simulink model "KalmanObserver_R2021b"  (R2021b)
settings: Solver=ode1  StartTime=0.0  StopTime=10  FixedStep=0.01  RelTol=1e-3
libraries: TcTargetLib x10
settings Model: SimulationMode=external  NumberOfSteps=50  PacingRate=0.280000  Creator=ATLabor  LastModifiedBy=Mergin
settings OptimizationCC: LocalBlockOutputs=off
settings RTWCC: Description=TwinCAT GRT Target  SystemTargetFile=TwinCatGrt.tlc  GenCodeOnly=on  TemplateMakefile=tcgrt_msbuild.tmf  TargetLang=C++
settings STFCustomTargetCC: TargetLangStandard=C++11 (ISO)  CombineOutputUpdateFcns=on  CPPClassGenCompliant=on  GRTInterface=off  SystemTargetFile=TwinCatGrt.tlc
settings GRTTargetCC: TargetLangStandard=C++11 (ISO)  ParMdlRefBuildCompliant=off  CompOptLevelCompliant=off  ConcurrentExecutionCompliant=off  MatFileLogging=off  UseToolchainInfoCompliant=off  ExtModeMexFile=TcExtModeClient

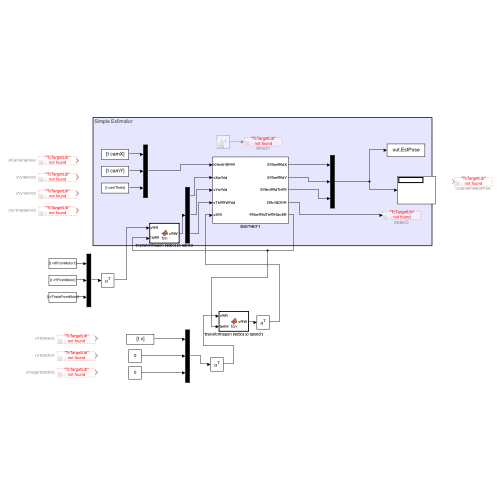
[thumbnail: Simulink's stored preview of the top-level diagram]
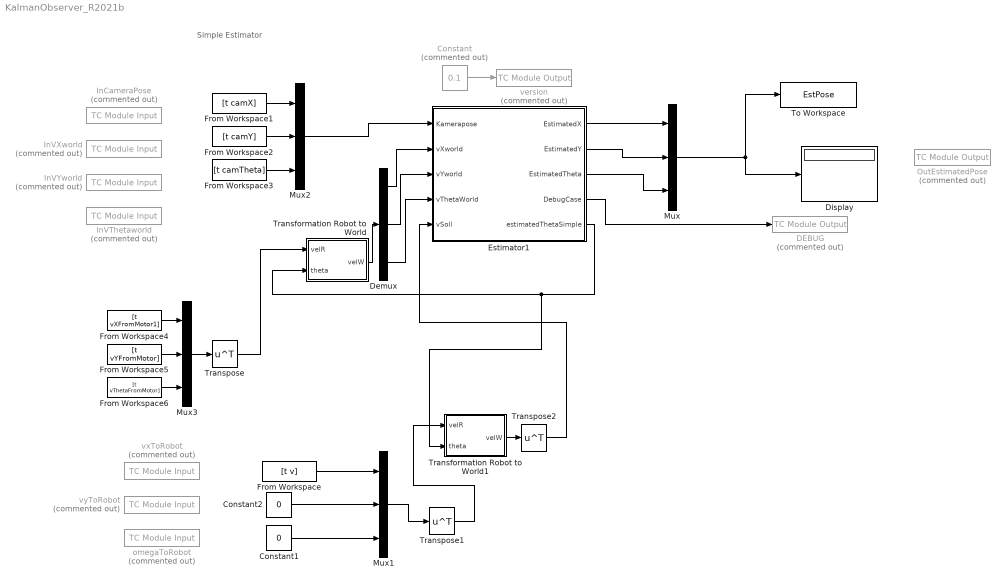
== system KalmanObserver_R2021b ==
  note: Simple Estimator
  Constant : Constant  Commented=on  Value=0.1
  Constant1 : Constant  Value=0
  Constant2 : Constant  Value=0
  DEBUG : TcTargetLib/TC Module Output  Commented=on  PortDataType=double  PortDim=1  SampleTime=-1  CodeGenConnectType=DataArea (OutputSrc)  DataTypeOverride=off
  Demux : Demux  Outputs=3
  Display : Display
  Estimator1 : Subsystem
  From Workspace : FromWorkspace  VariableName=[t v]  SampleTime=10e-3  OutputAfterFinalValue=Setting to zero
  From Workspace1 : FromWorkspace  VariableName=[t camX]  OutputAfterFinalValue=Holding final value
  From Workspace2 : FromWorkspace  VariableName=[t camY]  OutputAfterFinalValue=Holding final value
  From Workspace3 : FromWorkspace  VariableName=[t camTheta]  OutputAfterFinalValue=Holding final value
  From Workspace4 : FromWorkspace  VariableName=[t vXFromMotor1]  OutputAfterFinalValue=Setting to zero
  From Workspace5 : FromWorkspace  VariableName=[t vYFromMotor]  OutputAfterFinalValue=Setting to zero
  From Workspace6 : FromWorkspace  VariableName=[t vThetaFromMotor]  OutputAfterFinalValue=Setting to zero
  InCameraPose : TcTargetLib/TC Module Input  Commented=on  PortDataType=double  PortDim=3  Value=[0 0 0]  SampleTime=-1  CodeGenConnectType=DataArea (InputDst)  DataTypeOverride=on
  InVThetaworld : TcTargetLib/TC Module Input  Commented=on  PortDataType=double  PortDim=1  Value=0  SampleTime=-1  CodeGenConnectType=DataArea (InputDst)  DataTypeOverride=off
  InVXworld : TcTargetLib/TC Module Input  Commented=on  PortDataType=double  PortDim=1  Value=0  SampleTime=-1  CodeGenConnectType=DataArea (InputDst)  DataTypeOverride=off
  InVYworld : TcTargetLib/TC Module Input  Commented=on  PortDataType=double  PortDim=1  Value=0  SampleTime=-1  CodeGenConnectType=DataArea (InputDst)  DataTypeOverride=off
  Mux{,1..3} (4 alike) : Mux  Inputs=3
  OutEstimatedPose : TcTargetLib/TC Module Output  Commented=on  PortDataType=double  PortDim=3  SampleTime=-1  CodeGenConnectType=DataArea (OutputSrc)  DataTypeOverride=off
  To Workspace : ToWorkspace  VariableName=EstPose  SaveFormat=Timeseries  SampleTime=-1
  Transformation Robot to World : MATLAB Function  TreatAsAtomicUnit=on
  Transformation Robot to World1 : MATLAB Function  TreatAsAtomicUnit=on
  Transpose : Math  Operator=transpose  SaturateOnIntegerOverflow=on
  Transpose1 : Math  Operator=transpose  SaturateOnIntegerOverflow=on
  Transpose2 : Math  Operator=transpose  SaturateOnIntegerOverflow=on
  omegaToRobot : TcTargetLib/TC Module Input  Commented=on  PortDataType=double  PortDim=1  Value=0  SampleTime=-1  CodeGenConnectType=DataArea (InputDst)  DataTypeOverride=off
  version : TcTargetLib/TC Module Output  Commented=on  PortDataType=double  PortDim=1  SampleTime=-1  CodeGenConnectType=DataArea (OutputSrc)  DataTypeOverride=off
  vxToRobot : TcTargetLib/TC Module Input  Commented=on  PortDataType=double  PortDim=1  Value=0  SampleTime=-1  CodeGenConnectType=DataArea (InputDst)  DataTypeOverride=off
  vyToRobot : TcTargetLib/TC Module Input  Commented=on  PortDataType=double  PortDim=1  Value=0  SampleTime=-1  CodeGenConnectType=DataArea (InputDst)  DataTypeOverride=off
  wires:
  Estimator1/3(EstimatedTheta) -> Mux/3
  Constant/1 -> version/1
  Demux/2 -> Estimator1/3(vYworld)
  Estimator1/1(EstimatedX) -> Mux/1
  Estimator1/2(EstimatedY) -> Mux/2
  Demux/1 -> Estimator1/2(vXworld)
  Demux/3 -> Estimator1/4(vThetaWorld)
  Mux2/1 -> Estimator1/1(Kamerapose)
  Estimator1/4(DebugCase) -> DEBUG/1
  From Workspace/1 -> Mux1/1
  Constant1/1 -> Mux1/3
  Constant2/1 -> Mux1/2
  Mux1/1 -> Transpose1/1
  From Workspace1/1 -> Mux2/1
  From Workspace2/1 -> Mux2/2
  From Workspace3/1 -> Mux2/3
  From Workspace4/1 -> Mux3/1
  From Workspace5/1 -> Mux3/2
  From Workspace6/1 -> Mux3/3
  Mux3/1 -> Transpose/1
  Transformation Robot to World/1(velW) -> Demux/1
  Mux/1 -> To Workspace/1, Display/1
  Transpose/1 -> Transformation Robot to World/1(velR)
  Estimator1/5(estimatedThetaSimple) -> Transformation Robot to World1/2(theta), Transformation Robot to World/2(theta)
  Transpose2/1 -> Estimator1/5(vSoll)
  Transpose1/1 -> Transformation Robot to World1/1(velR)
  Transformation Robot to World1/1(velW) -> Transpose2/1

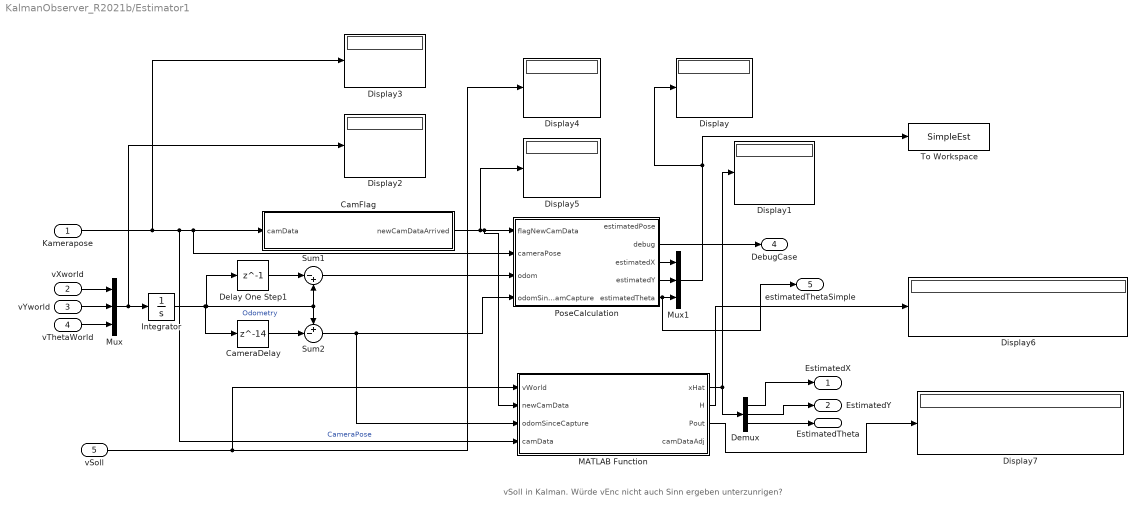
== system KalmanObserver_R2021b/Estimator1 ==
  note: vSoll in Kalman. Würde vEnc nicht auch Sinn ergeben unterzunrigen?
  Kamerapose : Inport
  vXworld : Inport  Port=2
  vYworld : Inport  Port=3
  vThetaWorld : Inport  Port=4
  vSoll : Inport  Port=5
  CamFlag : MATLAB Function  TreatAsAtomicUnit=on
  CameraDelay : Delay  DelayLength=14
  Delay One Step1 : Delay  DelayLength=1
  Demux : Demux  Outputs=3
  Display{,1..7} (8 alike) : Display
  Integrator : Integrator
  MATLAB Function : MATLAB Function  TreatAsAtomicUnit=on
  Mux : Mux  Inputs=3
  Mux1 : Mux  Inputs=3
  PoseCalculation : MATLAB Function  TreatAsAtomicUnit=on
  Sum1 : Sum  Inputs=|-+
  Sum2 : Sum  Inputs=+-|
  To Workspace : ToWorkspace  VariableName=SimpleEst  SaveFormat=Timeseries  SampleTime=-1
  EstimatedX : Outport
  EstimatedY : Outport  Port=2
  EstimatedTheta : Outport  Port=3
  DebugCase : Outport  Port=4
  estimatedThetaSimple : Outport  Port=5
  wires:
  vThetaWorld/1 -> Mux/3
  Sum2/1 -> MATLAB Function/3(odomSinceCapture), PoseCalculation/4(odomSinceCamCapture)
  vXworld/1 -> Mux/1
  Kamerapose/1 -> Display3/1, MATLAB Function/4(camData), PoseCalculation/2(cameraPose), CamFlag/1(camData)  "CameraPose"
  Integrator/1 -> Sum1/2, Sum2/1, Delay One Step1/1, CameraDelay/1  "Odometry"
  vYworld/1 -> Mux/2
  CamFlag/1(newCamDataArrived) -> Display5/1, MATLAB Function/2(newCamData), PoseCalculation/1(flagNewCamData)
  Delay One Step1/1 -> Sum1/1
  Sum1/1 -> PoseCalculation/3(odom)
  PoseCalculation/2(debug) -> DebugCase/1
  Demux/1 -> EstimatedX/1
  Mux/1 -> Display2/1, Integrator/1
  CameraDelay/1 -> Sum2/2
  MATLAB Function/1(xHat) -> Demux/1, Display1/1
  Demux/3 -> EstimatedTheta/1
  Demux/2 -> EstimatedY/1
  vSoll/1 -> Display4/1, MATLAB Function/1(vWorld)
  Mux1/1 -> To Workspace/1, Display/1
  PoseCalculation/3(estimatedX) -> Mux1/1
  PoseCalculation/4(estimatedY) -> Mux1/2
  PoseCalculation/5(estimatedTheta) -> estimatedThetaSimple/1, Mux1/3
  MATLAB Function/2(H) -> Display6/1
  MATLAB Function/3(Pout) -> Display7/1

== matlab function KalmanObserver_R2021b/Transformation Robot to World ==
  data: velR input; velW output size=[1 3]; theta input
function velW = fcn(velR, theta)
    TMat = [cos(theta)    -sin(theta)   0;
            sin(theta)    cos(theta)    0;
            0             0             1];
    velW = velR*transpose(TMat);
end

== matlab function KalmanObserver_R2021b/Estimator1/MATLAB Function ==
  settings: updateMethod=DISCRETE  sampleTime=10e-3
  data: vWorld input; xHat output; newCamData input; odomSinceCapture input; camData input; H output; Pout output; camDataAdj output
function [xHat, H, Pout, camDataAdj]= Kalman(vWorld, newCamData, odomSinceCapture, camData)

persistent xHatOld;
persistent P;

if isempty(xHatOld)
    xHatOld = [0; 0; 0];
    xHat = xHatOld;
end

if isempty(P)
    P = zeros(3,3);
end
camDataAdj =[0; 0; 0];
%% Systemparameter
A = [1 0 0;
     0 1 0;
     0 0 1];

taskTime = 10e-3; %10ms

B = [taskTime; taskTime; taskTime];

%C = [1 1 1];
C = eye(3);

R = [0.00127820524383046    -0.00144745069148629    1.57202639633006e-06;
    -0.00144745069148629    0.0142936660651043      -2.43008878392535e-05;
    1.57202639633006e-06    -2.43008878392535e-05	2.50703907504212e-07];

Q =[3.8635    0.4415   -0.0036;
    0.4415    9.3899   -0.0078;
   -0.0036   -0.0078    0.0001];

%% Prediction
xHatAp = A * xHatOld + B .* vWorld;
PAp = A * P * A' + Q;
xHat = xHatAp;
P = PAp;
%% Optimizing
%H = PAp * C' .* inv(C*PAp*C'+R);
H = PAp * inv(PAp+R);

%% Correction (only when new, valid Cam-Measurement)
if newCamData
    camDataAdj = camData + odomSinceCapture;
    xHat = xHatAp + H * (camDataAdj - C*xHatOld);  %normal Kalman Calculation
    %xHat = xHat + odomSinceCapture; % add odometrie difference since cameraMeasurement was taken to equalize cam delay
    P = PAp - H*C*PAp;
    %P = PAp - H*PAp;
end

xHatOld = xHat;
Pout = P;

== matlab function KalmanObserver_R2021b/Transformation Robot to World1 ==
  data: velR input; velW output size=[1 3]; theta input
function velW = fcn(velR, theta)
    TMat = [cos(theta)    -sin(theta)   0;
            sin(theta)    cos(theta)    0;
            0             0             1];
    velW = velR*transpose(TMat);
end

== matlab function KalmanObserver_R2021b/Estimator1/CamFlag ==
  settings: updateMethod=DISCRETE  sampleTime=10e-3
  data: camData input; newCamDataArrived output
function newCamDataArrived = fcn(camData)

persistent oldCamData

if isempty(oldCamData)
    oldCamData = [0 0 0]';
end

if camData ~= oldCamData %% && all(camData(1:2))   % all() prueft, ob x,y-Koordinate ungleich Null, um ungültige Kamerawerte zu entfernen. Kamerasystem sendet [0 0 0], wenn Fehler in Berechnung. Nur erste beiden Elemente pruefen, da Theta=0 zulaessig.
    if all(camData(1:2))
        newCamDataArrived = true;
    else
        newCamDataArrived = false;
    end
else
    newCamDataArrived = false;
    oldCamData = camData;
end
oldCamData = camData;

== matlab function KalmanObserver_R2021b/Estimator1/PoseCalculation ==
  settings: updateMethod=DISCRETE
  data: flagNewCamData input; cameraPose input; estimatedPose output; odom input; odomSinceCamCapture input; debug output; estimatedX output; estimatedY output; estimatedTheta output
function [estimatedPose, debug, estimatedX, estimatedY, estimatedTheta]= fcn(flagNewCamData, cameraPose, odom, odomSinceCamCapture)

% Variables
persistent estPoseOld

if isempty(estPoseOld)
    estPoseOld = [0 0 0]';
end

% Case 1: Camera Flag is set (New Cameradata) and CameraData is valid
if flagNewCamData == 1
    estimatedPose = cameraPose(1:3) + odomSinceCamCapture;   %OdomSinceCamCapture describes the pose changes since the camera captured the position because the camera data is delayed. in this time the robot drives further.
    estPoseOld = estimatedPose;
    debug = 1;

    % Case 2: No new Cameradata or invalid Cmeradata (integrate transformed velocities of
    % roboter in worldframe
else
    estimatedPose = estPoseOld + odom;
    estPoseOld = estimatedPose;  
    debug =2;
end

estimatedX = estimatedPose(1);
estimatedY = estimatedPose(2);
estimatedTheta = estimatedPose(3);
